simulink model "nonlinear_openloopObserver"  (R2021b)
settings: Solver=VariableStepAuto  StartTime=0.0  StopTime=40  RelTol=1e-3
undefined symbols (not defined in the file): A_obCx, B_obCx, C_obCx, Cx, D_obCx
settings Model: Creator=Anubhav Paras  LastModifiedBy=vanshika
settings SolverCC: AlgebraicLoopSolver=TrustRegion
settings DebuggingCC: SFMachineParentedDataDiag=warning

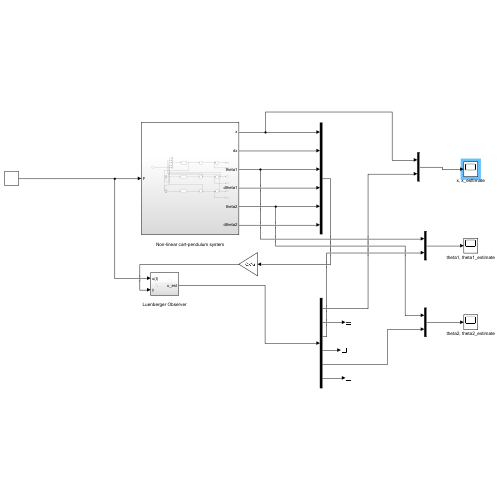
[thumbnail: Simulink's stored preview of the top-level diagram]
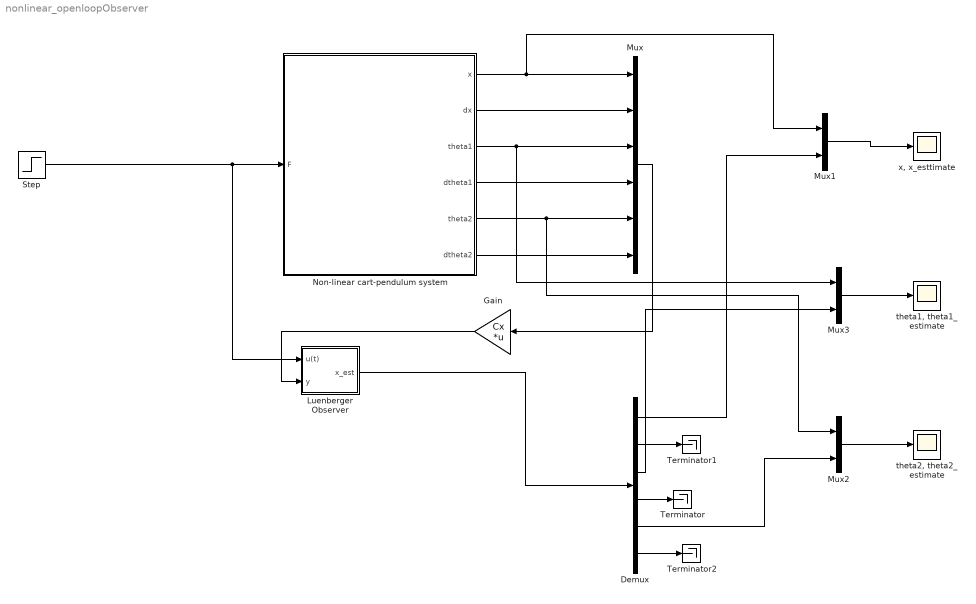
== system nonlinear_openloopObserver ==
  " Luenberger Observer" : Subsystem
  " Non-linear cart-pendulum system" : Subsystem
  Demux : Demux  Outputs=6
  Gain : Gain  Gain=Cx  Multiplication=Matrix(K*u)
  Mux : Mux  Inputs=6
  Mux1 : Mux  Inputs=2
  Mux2 : Mux  Inputs=2
  Mux3 : Mux  Inputs=2
  Step : Step  SampleTime=0
  Terminator : Terminator
  Terminator1 : Terminator
  Terminator2 : Terminator
  "theta1, theta1_estimate" : Scope
  "theta2, theta2_estimate" : Scope
  "x, x_esttimate" : Scope
  wires:
  Demux/3 -> Mux3/2
  Mux/1 -> Gain/1
  Gain/1 -> " Luenberger Observer"/2(y)
  " Non-linear cart-pendulum system"/6(dtheta2) -> Mux/6
  " Non-linear cart-pendulum system"/1(x) -> Mux/1, Mux1/1
  " Non-linear cart-pendulum system"/4(dtheta1) -> Mux/4
  " Non-linear cart-pendulum system"/3(theta1) -> Mux/3, Mux3/1
  " Non-linear cart-pendulum system"/5(theta2) -> Mux/5, Mux2/1
  " Non-linear cart-pendulum system"/2(dx) -> Mux/2
  Mux1/1 -> "x, x_esttimate"/1
  Mux3/1 -> "theta1, theta1_estimate"/1
  Demux/5 -> Mux2/2
  Mux2/1 -> "theta2, theta2_estimate"/1
  " Luenberger Observer"/1(x_est) -> Demux/1
  Demux/1 -> Mux1/2
  Step/1 -> " Non-linear cart-pendulum system"/1(F), " Luenberger Observer"/1(u(t))
  Demux/4 -> Terminator/1
  Demux/2 -> Terminator1/1
  Demux/6 -> Terminator2/1

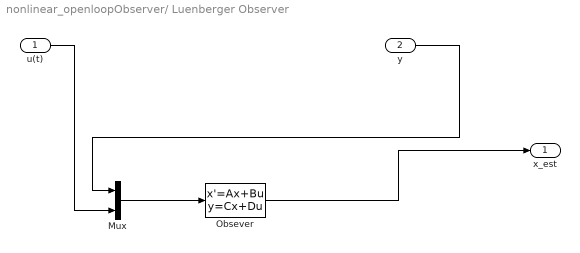
== system nonlinear_openloopObserver/ Luenberger Observer ==
  u(t) : Inport
  y : Inport  Port=2
  Mux : Mux  Inputs=2
  "Obsever " : StateSpace  A=A_obCx  B=B_obCx  C=C_obCx  D=D_obCx  InitialCondition=0
  x_est : Outport
  wires:
  Mux/1 -> "Obsever "/1
  "Obsever "/1 -> x_est/1
  y/1 -> Mux/1
  u(t)/1 -> Mux/2

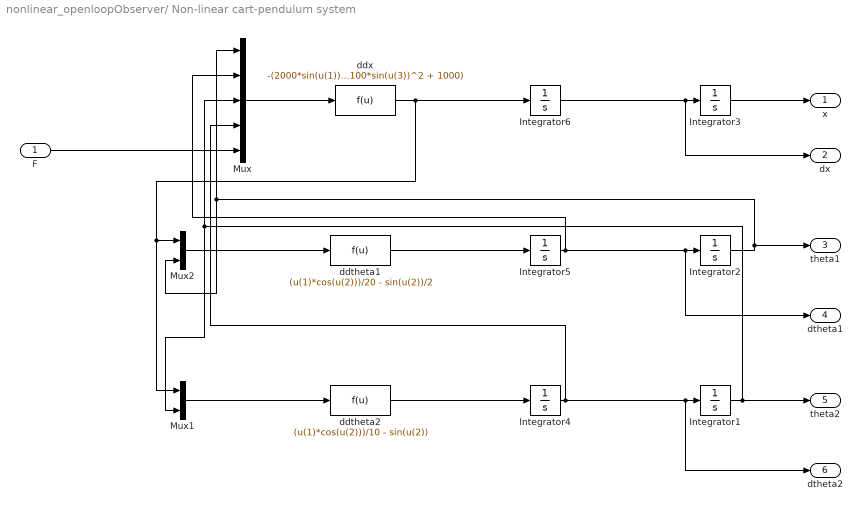
== system nonlinear_openloopObserver/ Non-linear cart-pendulum system ==
  F : Inport
  Integrator1 : Integrator  InitialCondition=0.1
  Integrator2 : Integrator  InitialCondition=0.1
  Integrator3 : Integrator  InitialCondition=0.5
  Integrator4 : Integrator
  Integrator5 : Integrator
  Integrator6 : Integrator
  Mux : Mux  Inputs=5
  Mux1 : Mux  Inputs=2
  Mux2 : Mux  Inputs=2
  ddtheta1 : Fcn  Expr=(u(1)*cos(u(2)))/20 - sin(u(2))/2
  ddtheta2 : Fcn  Expr=(u(1)*cos(u(2)))/10 - sin(u(2))
  ddx : Fcn  Expr=-(2000*sin(u(1))*u(2)^2 + 1000*sin(u(3))*u(4)^2 - u(5) + 1000*cos(u(1))*sin(u(1)) - 1000*cos(u(3))*sin(u(3)))/(100*sin(u(1))^2 + 100*sin(u(3))^2 + 1000)
  x : Outport
  dx : Outport  Port=2
  theta1 : Outport  Port=3
  dtheta1 : Outport  Port=4
  theta2 : Outport  Port=5
  dtheta2 : Outport  Port=6
  wires:
  ddtheta2/1 -> Integrator4/1
  ddx/1 -> Mux1/1, Mux2/1, Integrator6/1
  Integrator6/1 -> dx/1, Integrator3/1
  Mux1/1 -> ddtheta2/1
  Integrator5/1 -> Mux/2, dtheta1/1, Integrator2/1
  Mux/1 -> ddx/1
  Integrator1/1 -> theta2/1, Mux1/2, Mux/3
  Integrator2/1 -> theta1/1, Mux2/2, Mux/1
  ddtheta1/1 -> Integrator5/1
  Integrator4/1 -> Mux/4, dtheta2/1, Integrator1/1
  Mux2/1 -> ddtheta1/1
  Integrator3/1 -> x/1
  F/1 -> Mux/5
